simulink model "ModeloTanques"  (R2020a)
settings: Solver=ode45  StartTime=0.0  StopTime=200  RelTol=1e-3  EnableMultiTasking=on
libraries: simulink x6, fuzblock x1
settings Model: Creator=MeneghettiAir  LastModifiedBy=barbosa
settings DataIOCC: LimitDataPoints=on  SaveFormat=Array  ReturnWorkspaceOutputs=off
settings OptimizationCC: LifeSpan=inf
settings DebuggingCC: SolverPrmCheckMsg=warning  SFUnexpectedBacktrackingDiag=warning  SFNoUnconditionalDefaultTransitionDiag=warning  SFExecutionAtInitializationDiag=none  ArithmeticOperatorsInVariantConditions=warning
settings HardwareCC: ProdBitPerPointer=32  ProdBitPerSizeT=32  ProdBitPerPtrDiffT=32  ProdLargestAtomicFloat=None  ProdIntDivRoundTo=Undefined  ProdEndianess=Unspecified  ProdWordSize=32  ProdHWDeviceType=32-bit Generic
settings ModelReferenceCC: PropagateSignalLabelsOutOfModel=off
settings SFSimCC: SimUseLocalCustomCode=off  CustomCodeUndefinedFunction=UseInterfaceOnly
settings RTWCC: RTWUseLocalCustomCode=off
settings CodeAppCC: StateflowObjectComments=on
settings GRTTargetCC: TargetLangStandard=C89/C90 (ANSI)
settings ConfigComp: CovMetricSettings=dw  CovHtmlReporting=on  CovSaveCumulativeToWorkspaceVar=on  CovSaveSingleToWorkspaceVar=on  CovExternalEMLEnable=off  CovSFcnEnable=off

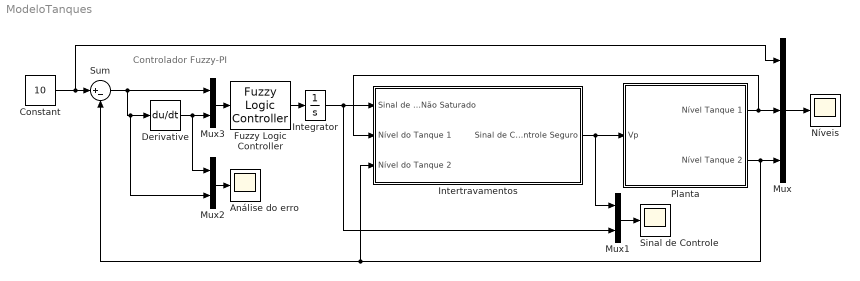
== system ModeloTanques ==
  note: Controlador Fuzzy-PI
  Análise do erro : Scope
  Constant : Constant  Value=10
  Derivative : Derivative
  Fuzzy Logic Controller : fuzblock/Fuzzy Logic  Controller  FIS="\"fis.fis\""  OutputSampleNumber=101  DataType=double  FuzzifiedInputs=off  RuleFiringStrengths=off  RuleOutputs=off  AggregatedOutputs=off  SimulateUsing=Interpreted execution  OutOfRangeInputValueMessage=warning  NoRuleFiredMessage=warning  EmptyOutputFuzzySetMessage=warning
  Integrator : Integrator
  Intertravamentos : Subsystem
  Mux : Mux  Inputs=3
  Mux1 : Mux  Inputs=2
  Mux2 : Mux  Inputs=2
  Mux3 : Mux  Inputs=2
  Níveis : Scope
  Planta : Subsystem
  Sinal de Controle : Scope
  Sum : Sum  Inputs=|+-
  wires:
  Planta/1(Nível Tanque 1) -> Intertravamentos/2(Nível do Tanque 1), Mux/2
  Planta/2(Nível Tanque 2) -> Mux/3, Sum/2, Intertravamentos/3(Nível do Tanque 2)
  Mux/1 -> Níveis/1
  Constant/1 -> Sum/1, Mux/1
  Mux1/1 -> Sinal de Controle/1
  Mux2/1 -> Análise do erro/1
  Derivative/1 -> Mux2/1, Mux3/2
  Sum/1 -> Mux3/1, Mux2/2, Derivative/1
  Intertravamentos/1(Sinal de Controle Seguro) -> Mux1/1, Planta/1(Vp)
  Mux3/1 -> Fuzzy Logic Controller/1
  Fuzzy Logic Controller/1 -> Integrator/1
  Integrator/1 -> Mux1/2, Intertravamentos/1(Sinal de Controle Não Saturado)

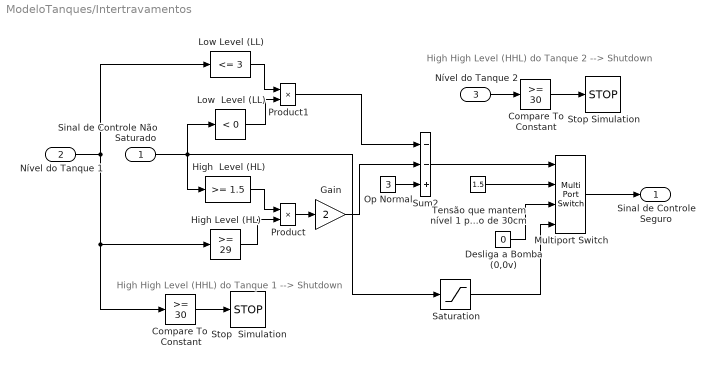
== system ModeloTanques/Intertravamentos ==
  note: High High Level (HHL) do Tanque 2 --> Shutdown
  note: High High Level (HHL) do Tanque 1 --> Shutdown
  Sinal de Controle Não Saturado : Inport
  Nível do Tanque 1 : Inport  Port=2
  Nível do Tanque 2 : Inport  Port=3
  Compare To  Constant : simulink/Logic and Bit Operations/Compare To Constant  relop=>=  const=30  OutDataTypeStr=boolean
  Compare To Constant : simulink/Logic and Bit Operations/Compare To Constant  relop=>=  const=30  OutDataTypeStr=boolean
  Desliga a Bomba (0,0v) : Constant  Value=0
  Gain : Gain  Gain=2
  High  Level (HL) : simulink/Logic and Bit Operations/Compare To Constant  relop=>=  const=1.5  OutDataTypeStr=uint8
  "High Level (HL)   " : simulink/Logic and Bit Operations/Compare To Constant  relop=>=  const=29  OutDataTypeStr=uint8
  Low  Level (LL) : simulink/Logic and Bit Operations/Compare To Constant  relop=<  const=0  OutDataTypeStr=uint8
  Low Level (LL) : simulink/Logic and Bit Operations/Compare To Constant  relop=<=  const=3  OutDataTypeStr=uint8
  Multiport Switch : MultiPortSwitch
  Op Normal : Constant  Value=3
  Product : Product
  Product1 : Product
  Saturation : Saturate  UpperLimit=4  LowerLimit=-4
  Stop  Simulation : Stop
  Stop Simulation : Stop
  Sum2 : Sum  Inputs=--+
  Tensão que mantem nível 1 próximo de 30cm : Constant  Value=1.5
  Sinal de Controle Seguro : Outport
  wires:
  Sinal de Controle Não Saturado/1 -> Saturation/1, Low  Level (LL)/1, High  Level (HL)/1
  Desliga a Bomba (0,0v)/1 -> Multiport Switch/3
  Tensão que mantem nível 1 próximo de 30cm/1 -> Multiport Switch/2
  Saturation/1 -> Multiport Switch/4
  Sum2/1 -> Multiport Switch/1
  Multiport Switch/1 -> Sinal de Controle Seguro/1
  Nível do Tanque 1/1 -> Low Level (LL)/1, Compare To  Constant/1, "High Level (HL)   "/1
  High  Level (HL)/1 -> Product/1
  "High Level (HL)   "/1 -> Product/2
  Low Level (LL)/1 -> Product1/1
  Low  Level (LL)/1 -> Product1/2
  Product1/1 -> Sum2/1
  Op Normal/1 -> Sum2/3
  Product/1 -> Gain/1
  Gain/1 -> Sum2/2
  Compare To Constant/1 -> Stop Simulation/1
  Nível do Tanque 2/1 -> Compare To Constant/1
  Compare To  Constant/1 -> Stop  Simulation/1

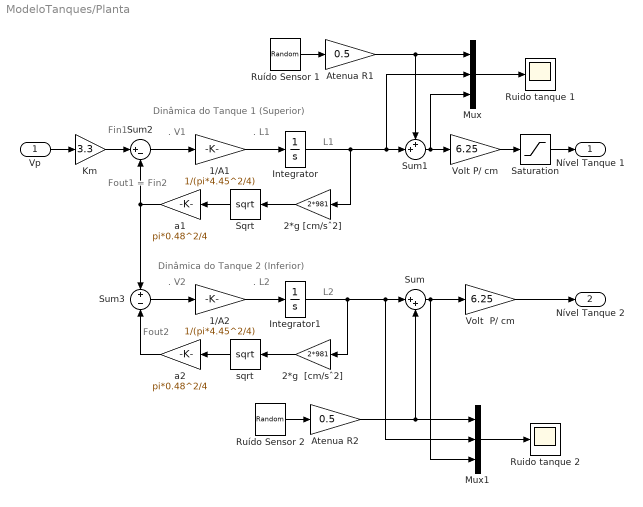
== system ModeloTanques/Planta ==
  note: Dinâmica do Tanque 1 (Superior)
  note: L1
  note: Fin1
  note: Fout1
      | =
      | Fin2
  note: .
      | L1
  note: .
      | V1
  note: L2
  note: Fout2
  note: .
      | L2
  note: .
      | V2
  note: Dinâmica do Tanque 2 (Inferior)
  Vp : Inport
  1/A1 : Gain  Gain=1/(pi*4.45^2/4)
  1/A2 : Gain  Gain=1/(pi*4.45^2/4)
  2*g  [cm/sˆ2] : Gain  Gain=2*981
  2*g [cm/sˆ2] : Gain  Gain=2*981
  Atenua R1 : Gain  Gain=0.5
  Atenua R2 : Gain  Gain=0.5
  Integrator : Integrator  LimitOutput=on  UpperSaturationLimit=32  LowerSaturationLimit=0
  Integrator1 : Integrator  LimitOutput=on  UpperSaturationLimit=32  LowerSaturationLimit=0
  Km : Gain  Gain=3.3
  Mux : Mux  Inputs=3
  Mux1 : Mux  Inputs=3
  Ruido tanque 1 : Scope
  Ruido tanque 2 : Scope
  Ruído Sensor 1 : UniformRandomNumber  Minimum=-0.01  Maximum=0.01  Seed=round(rand(1)*100)  SampleTime=0.5
  Ruído Sensor 2 : UniformRandomNumber  Minimum=-0.02  Maximum=0.02  Seed=round(rand(1)*100)  SampleTime=0.5
  Saturation : Saturate  UpperLimit=35  LowerLimit=-2
  Sqrt : Sqrt  SaturateOnIntegerOverflow=on
  Sum : Sum  Inputs=|++
  Sum1 : Sum  Inputs=++|
  Sum2 : Sum  Inputs=|+-
  Sum3 : Sum  Inputs=+-
  Volt  P/ cm : Gain  Gain=6.25
  Volt P/ cm : Gain  Gain=6.25
  a1 : Gain  Gain=pi*0.48^2/4
  a2 : Gain  Gain=pi*0.48^2/4
  sqrt : Sqrt  SaturateOnIntegerOverflow=on
  Nível Tanque 1 : Outport
  Nível Tanque 2 : Outport  Port=2
  wires:
  Vp/1 -> Km/1
  Integrator/1 -> 2*g [cm/sˆ2]/1, Mux/2, Sum1/2
  Volt P/ cm/1 -> Saturation/1
  Volt  P/ cm/1 -> Nível Tanque 2/1
  Sum/1 -> Mux1/3, Volt  P/ cm/1
  Ruído Sensor 2/1 -> Atenua R2/1
  Sum1/1 -> Mux/3, Volt P/ cm/1
  Ruído Sensor 1/1 -> Atenua R1/1
  Mux/1 -> Ruido tanque 1/1
  Mux1/1 -> Ruido tanque 2/1
  Saturation/1 -> Nível Tanque 1/1
  Atenua R1/1 -> Mux/1, Sum1/1
  Atenua R2/1 -> Sum/2, Mux1/1
  2*g [cm/sˆ2]/1 -> Sqrt/1
  Sqrt/1 -> a1/1
  Km/1 -> Sum2/1
  a1/1 -> Sum2/2, Sum3/1
  Sum2/1 -> 1/A1/1
  1/A1/1 -> Integrator/1
  Integrator1/1 -> 2*g  [cm/sˆ2]/1, Mux1/2, Sum/1
  2*g  [cm/sˆ2]/1 -> sqrt/1
  sqrt/1 -> a2/1
  Sum3/1 -> 1/A2/1
  1/A2/1 -> Integrator1/1
  a2/1 -> Sum3/2
